simulink library "CTRL_LO_ST1_YAWTRQSUM"  (R2023b)
settings: Solver=VariableStepAuto  StartTime=0.0  StopTime=10.0  RelTol=1e-3
settings Model: Creator=blatak  LastModifiedBy=blatak

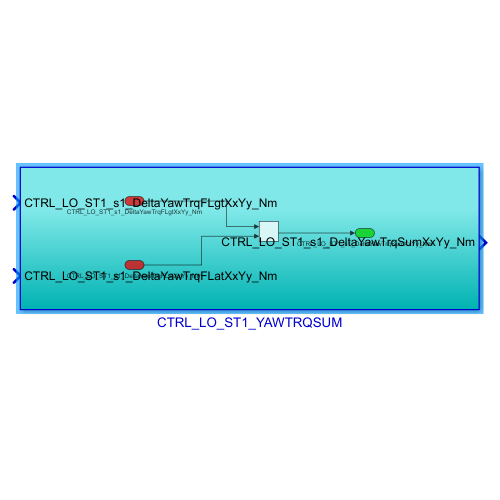
[thumbnail: Simulink's stored preview of the top-level diagram]
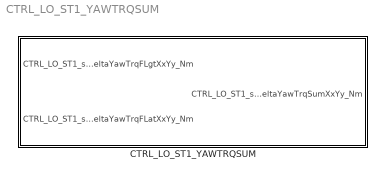
== system CTRL_LO_ST1_YAWTRQSUM ==
  CTRL_LO_ST1_YAWTRQSUM : Subsystem

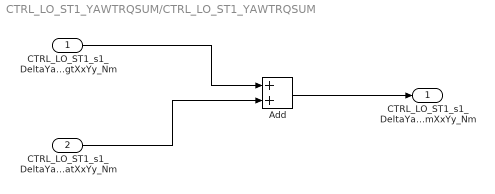
== system CTRL_LO_ST1_YAWTRQSUM/CTRL_LO_ST1_YAWTRQSUM ==
  CTRL_LO_ST1_s1_DeltaYawTrqFLgtXxYy_Nm : Inport
  CTRL_LO_ST1_s1_DeltaYawTrqFLatXxYy_Nm : Inport  Port=2
  Add : Sum
  CTRL_LO_ST1_s1_DeltaYawTrqSumXxYy_Nm : Outport
  wires:
  CTRL_LO_ST1_s1_DeltaYawTrqFLatXxYy_Nm/1 -> Add/2
  CTRL_LO_ST1_s1_DeltaYawTrqFLgtXxYy_Nm/1 -> Add/1
  Add/1 -> CTRL_LO_ST1_s1_DeltaYawTrqSumXxYy_Nm/1
